simulink model "Ford_T3T6_ArchCnctnDigrm"  (R2016b)
settings: Solver=FixedStepDiscrete  StartTime=0.0  StopTime=10.0  RelTol=1e-3  EnableMultiTasking=on
libraries: canmsglib x15
(part 12 of 15)

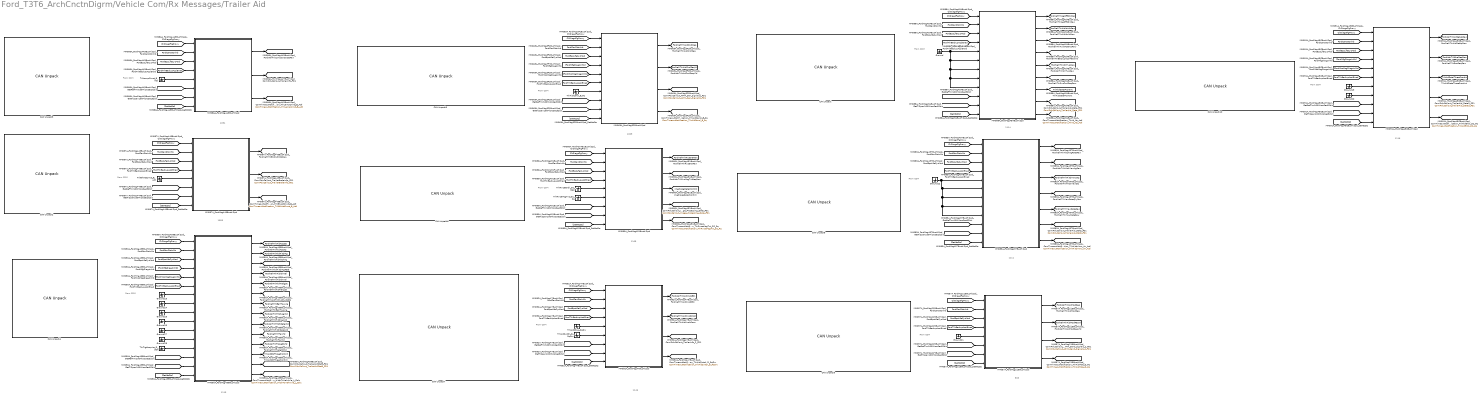
== system Ford_T3T6_ArchCnctnDigrm/Vehicle Com/Rx Messages/Trailer Aid ==
  note: 1116
  note: 533
  note: 1111
  note: 1114
  note: 1146
  note: 1105
  note: 1009
  note: 1113
  note: 1093
  note: 1091
  note: From COM
  note: From COM
  note: From COM
  note: From COM
  note: From COM
  note: From COM
  note: From COM
  note: From COM
  note: From COM
  note: From COM
  CAN Unpack : canmsglib/CAN Unpack  CANdbFile=C:\Users\nz3503\Desktop\Ford Architecture\FD1_CAN_P702_GASDHEV_MY21_V04.dbc  MsgList=TrailerAid_Data_FD1  MsgName=TrailerAid_Data_FD1  MsgIDType=Standard (11-bit identifier)  MsgIdentifier=1114  MsgLength=8  SignalInfo=TrailCtlSwtch_B_Stat2$16$1$2$2$1$0$1$0$0$1$#TrlBrkInitOut_D_Rq$59$2$2$2$1$0$1$0$0$3$#TrlrAidEnbl_D_Rq$13$2$2$2$1$0$1$0$0$3$#TrlrAidSetup_D_Rq$57$2$2$2$1$0$1$0$0$3$#TrlrAnOffstDir_D_Mem$61$2$2$2$1$0$1$0$0$3$#TrlrAnOffst_An_Mem$63$9$2$2$1$0$1.000000e-01$0$0$5.110000e+01$#TrlrAxleToBmpr_L_Actl$15$9$2$2$1$0$2.540000e-02$0$0$1.297940e+01$#TrlrBallToBmpr_L_Actl$17$7$2$2$1$0$1.270000e-02$0$0$1.612900e+00$#TrlrIdType_D_Stat$32$2$2$2$1$0$1$0$0$3$#TrlrId_No_Actl$9$4$2$2$1$0$1$0$0$15$#TrlrRvrseCancl_B_Rq$8$1$2$2$1$0$1$0$0$1$#TrlrTrgtOffst_L_Actl$41$7$2$2$1$0$1.270000e-02$0$0$1.612900e+00$#TrlrTrgtPtrnId_No_Mem$34$6$2$2$1$0$1$0$0$63$#TrlrTrgtToBmpr_L_Actl$25$7$2$2$1$0$1.270000e-02$0$0$1.612900e+00$#  NSignals=14  IDPort=off  TimestampPort=off  ErrorPort=off  RemotePort=off  LengthPort=off  StatusPort=off  StartBits=str2num('[int32(16);int32(59);int32(13);int32(57);int32(61);int32(63);int32(15);int32(17);int32(32);int32(9);int32(8);int32(41);int32(34);int32(25)]')  SignalSizes=str2num('[int32(1);int32(2);int32(2);int32(2);int32(2);int32(9);int32(9);int32(7);int32(2);int32(4);int32(1);int32(7);int32(6);int32(7)]')  ByteOrders=str2num('[int32(2);int32(2);int32(2);int32(2);int32(2);int32(2);int32(2);int32(2);int32(2);int32(2);int32(2);int32(2);int32(2);int32(2)]')  DataTypes=str2num('[int32(2);int32(2);int32(2);int32(2);int32(2);int32(2);int32(2);int32(2);int32(2);int32(2);int32(2);int32(2);int32(2);int32(2)]')  MultiplexTypes=str2num('[int32(1);int32(1);int32(1);int32(1);int32(1);int32(1);int32(1);int32(1);int32(1);int32(1);int32(1);int32(1);int32(1);int32(1)]')  MultiplexValues=str2num('[double(0);double(0);double(0);double(0);double(0);double(0);double(0);double(0);double(0);double(0);double(0);double(0);double(0);double(0)]')  Factors=str2num('[double(1);double(1);double(1);double(1);double(1);double(1.000000e-01);double(2.540000e-02);double(1.270000e-02);double(1);double(1);double(1);double(1.270000e-02);double(1);double(1.270000e-02)]')  Offsets=str2num('[double(0);double(0);double(0);double(0);double(0);double(0);double(0);double(0);double(0);double(0);double(0);double(0);double(0);double(0)]')  Minimums=str2num('[double(0);double(0);double(0);double(0);double(0);double(0);double(0);double(0);double(0);double(0);double(0);double(0);double(0);double(0)]')  Maximums=str2num('[double(1);double(3);double(3);double(3);double(3);double(5.110000e+01);double(1.297940e+01);double(1.612900e+00);double(3);double(15);double(1);double(1.612900e+00);double(63);double(1.612900e+00)]')
      settings: DataFormat=CANdb specified signals
  CAN Unpack10 : canmsglib/CAN Unpack  CANdbFile=C:\Users\nz3503\Desktop\Ford Architecture\FD1_CAN_P702_GASDHEV_MY21_V04.dbc  MsgList=TrailerAid_Data3_FD1  MsgName=TrailerAid_Data3_FD1  MsgIDType=Standard (11-bit identifier)  MsgIdentifier=1116  MsgLength=8  SignalInfo=TrlrAidEnbl_D2_Rq$5$3$2$2$1$0$1$0$0$7$#TrlrAidSetup_D2_Rq$1$4$2$2$1$0$1$0$0$15$#  NSignals=2  IDPort=off  TimestampPort=off  ErrorPort=off  RemotePort=off  LengthPort=off  StatusPort=off  StartBits=str2num('[int32(5);int32(1)]')  SignalSizes=str2num('[int32(3);int32(4)]')  ByteOrders=str2num('[int32(2);int32(2)]')  DataTypes=str2num('[int32(2);int32(2)]')  MultiplexTypes=str2num('[int32(1);int32(1)]')  MultiplexValues=str2num('[double(0);double(0)]')  Factors=str2num('[double(1);double(1)]')  Offsets=str2num('[double(0);double(0)]')  Minimums=str2num('[double(0);double(0)]')  Maximums=str2num('[double(7);double(15)]')
      settings: DataFormat=CANdb specified signals
  CAN Unpack2 : canmsglib/CAN Unpack  CANdbFile=C:\Users\nz3503\Desktop\Ford Architecture\FD1_CAN_P702_GASDHEV_MY21_V04.dbc  MsgList=TrailerBrakeInfo_FD1  MsgName=TrailerBrakeInfo_FD1  MsgIDType=Standard (11-bit identifier)  MsgIdentifier=1093  MsgLength=8  SignalInfo=StopLamp_B_RqTrlrBrk$7$1$2$2$1$0$1$0$0$1$#TrlBrkInitOut_D_Stat$9$2$2$2$1$0$1$0$0$3$#TrlrBrkActCirct_B_Falt$1$1$2$2$1$0$1$0$0$1$#TrlrBrkActCnnct_B_Actl$6$1$2$2$1$0$1$0$0$1$#TrlrBrkCtl_B_Falt$4$1$2$2$1$0$1$0$0$1$#TrlrBrkDcnnt_B_Actl$5$1$2$2$1$0$1$0$0$1$#TrlrBrkDsply_B_Rq$3$1$2$2$1$0$1$0$0$1$#TrlrBrkGain_No_Actl$11$5$2$2$1$0$5.000000e-01$0$0$1.550000e+01$#TrlrBrkMde_D_Actl$2$1$2$2$1$0$1$0$0$1$#TrlrBrkOut_No_Dsply$20$4$2$2$1$0$1$0$0$15$#  NSignals=10  IDPort=off  TimestampPort=off  ErrorPort=off  RemotePort=off  LengthPort=off  StatusPort=off  StartBits=str2num('[int32(7);int32(9);int32(1);int32(6);int32(4);int32(5);int32(3);int32(11);int32(2);int32(20)]')  SignalSizes=str2num('[int32(1);int32(2);int32(1);int32(1);int32(1);int32(1);int32(1);int32(5);int32(1);int32(4)]')  ByteOrders=str2num('[int32(2);int32(2);int32(2);int32(2);int32(2);int32(2);int32(2);int32(2);int32(2);int32(2)]')  DataTypes=str2num('[int32(2);int32(2);int32(2);int32(2);int32(2);int32(2);int32(2);int32(2);int32(2);int32(2)]')  MultiplexTypes=str2num('[int32(1);int32(1);int32(1);int32(1);int32(1);int32(1);int32(1);int32(1);int32(1);int32(1)]')  MultiplexValues=str2num('[double(0);double(0);double(0);double(0);double(0);double(0);double(0);double(0);double(0);double(0)]')  Factors=str2num('[double(1);double(1);double(1);double(1);double(1);double(1);double(1);double(5.000000e-01);double(1);double(1)]')  Offsets=str2num('[double(0);double(0);double(0);double(0);double(0);double(0);double(0);double(0);double(0);double(0)]')  Minimums=str2num('[double(0);double(0);double(0);double(0);double(0);double(0);double(0);double(0);double(0);double(0)]')  Maximums=str2num('[double(1);double(3);double(1);double(1);double(1);double(1);double(1);double(1.550000e+01);double(1);double(15)]')
      settings: DataFormat=CANdb specified signals
  CAN Unpack3 : canmsglib/CAN Unpack  CANdbFile=C:\Users\nz3503\Desktop\Ford Architecture\FD1_CAN_P702_GASDHEV_MY21_V04.dbc  MsgList=TrailerInfo_FD1  MsgName=TrailerInfo_FD1  MsgIDType=Standard (11-bit identifier)  MsgIdentifier=1091  MsgLength=8  SignalInfo=CamraRearOn_D2_Stat2$9$3$2$2$1$0$1$0$0$7$#ParkLampTrlrOut_B_Stat$15$1$2$2$1$0$1$0$0$1$#PoliceAux1Lamp_B_Rq2$8$1$2$2$1$0$1$0$0$1$#PoliceAux2Lamp_B_Rq2$23$1$2$2$1$0$1$0$0$1$#PoliceAux3Lamp_B_Rq2$22$1$2$2$1$0$1$0$0$1$#PoliceAux4Lamp_B_Rq2$21$1$2$2$1$0$1$0$0$1$#StopLampTrlrOut_B_Stat$0$1$2$2$1$0$1$0$0$1$#TowBarMsgTxt_D_Rq$12$3$2$2$1$0$1$0$0$7$#TrlrBattChrg_D_Stat$1$2$2$2$1$0$1$0$0$3$#TrlrLampCnnct_B_Actl$7$1$2$2$1$0$1$0$0$1$#TrlrLampCtl_D_Stat$3$2$2$2$1$0$1$0$0$3$#TurnLampTrlrRl_B_Stat$6$1$2$2$1$0$1$0$0$1$#TurnLampTrlrRr_B_Stat$5$1$2$2$1$0$1$0$0$1$#  NSignals=13  IDPort=off  TimestampPort=off  ErrorPort=off  RemotePort=off  LengthPort=off  StatusPort=off  StartBits=str2num('[int32(9);int32(15);int32(8);int32(23);int32(22);int32(21);int32(0);int32(12);int32(1);int32(7);int32(3);int32(6);int32(5)]')  SignalSizes=str2num('[int32(3);int32(1);int32(1);int32(1);int32(1);int32(1);int32(1);int32(3);int32(2);int32(1);int32(2);int32(1);int32(1)]')  ByteOrders=str2num('[int32(2);int32(2);int32(2);int32(2);int32(2);int32(2);int32(2);int32(2);int32(2);int32(2);int32(2);int32(2);int32(2)]')  DataTypes=str2num('[int32(2);int32(2);int32(2);int32(2);int32(2);int32(2);int32(2);int32(2);int32(2);int32(2);int32(2);int32(2);int32(2)]')  MultiplexTypes=str2num('[int32(1);int32(1);int32(1);int32(1);int32(1);int32(1);int32(1);int32(1);int32(1);int32(1);int32(1);int32(1);int32(1)]')  MultiplexValues=str2num('[double(0);double(0);double(0);double(0);double(0);double(0);double(0);double(0);double(0);double(0);double(0);double(0);double(0)]')  Factors=str2num('[double(1);double(1);double(1);double(1);double(1);double(1);double(1);double(1);double(1);double(1);double(1);double(1);double(1)]')  Offsets=str2num('[double(0);double(0);double(0);double(0);double(0);double(0);double(0);double(0);double(0);double(0);double(0);double(0);double(0)]')  Minimums=str2num('[double(0);double(0);double(0);double(0);double(0);double(0);double(0);double(0);double(0);double(0);double(0);double(0);double(0)]')  Maximums=str2num('[double(7);double(1);double(1);double(1);double(1);double(1);double(1);double(7);double(3);double(1);double(3);double(1);double(1)]')
      settings: DataFormat=CANdb specified signals
  CAN Unpack4 : canmsglib/CAN Unpack  CANdbFile=C:\Users\nz3503\Desktop\Ford Architecture\FD1_CAN_P702_GASDHEV_MY21_V04.dbc  MsgList=TrailerAid_Stat3_FD1  MsgName=TrailerAid_Stat3_FD1  MsgIDType=Standard (11-bit identifier)  MsgIdentifier=1113  MsgLength=8  SignalInfo=HitchToTrlrAxle_L_Calc2$23$9$2$2$1$0$2.540000e-02$0$0$1.297940e+01$#HitchToVehAxle_L_Calc$0$8$2$2$1$0$1.270000e-02$-5.080000e-01$-5.080000e-01$2.717800e+00$#TrlrAidTrgtId_No_Actl$43$5$2$2$1$0$1$0$0$31$#TrlrAid_An3_Actl$34$11$2$2$1$0$1.250000e-01$-90$-90$1.657500e+02$#TrlrAid_AnRate2_Actl$29$10$2$2$1$0$1.250000e-01$-50$-50$7.775000e+01$#TrlrAid_D2_Stat$52$4$2$2$1$0$1$0$0$15$#TrlrAnCalib_B_Complt$40$1$2$2$1$0$1$0$0$1$#TrlrAnOffstDir_D_Calc$32$2$2$2$1$0$1$0$0$3$#TrlrAnOffst_An_Calc$56$9$2$2$1$0$1.000000e-01$0$0$5.110000e+01$#TrlrRvrse_D_Stat$41$2$2$2$1$0$1$0$0$3$#TrlrTrgtAcquire_D_Stat$49$3$2$2$1$0$1$0$0$7$#  NSignals=11  IDPort=off  TimestampPort=off  ErrorPort=off  RemotePort=off  LengthPort=off  StatusPort=off  StartBits=str2num('[int32(23);int32(0);int32(43);int32(34);int32(29);int32(52);int32(40);int32(32);int32(56);int32(41);int32(49)]')  SignalSizes=str2num('[int32(9);int32(8);int32(5);int32(11);int32(10);int32(4);int32(1);int32(2);int32(9);int32(2);int32(3)]')  ByteOrders=str2num('[int32(2);int32(2);int32(2);int32(2);int32(2);int32(2);int32(2);int32(2);int32(2);int32(2);int32(2)]')  DataTypes=str2num('[int32(2);int32(2);int32(2);int32(2);int32(2);int32(2);int32(2);int32(2);int32(2);int32(2);int32(2)]')  MultiplexTypes=str2num('[int32(1);int32(1);int32(1);int32(1);int32(1);int32(1);int32(1);int32(1);int32(1);int32(1);int32(1)]')  MultiplexValues=str2num('[double(0);double(0);double(0);double(0);double(0);double(0);double(0);double(0);double(0);double(0);double(0)]')  Factors=str2num('[double(2.540000e-02);double(1.270000e-02);double(1);double(1.250000e-01);double(1.250000e-01);double(1);double(1);double(1);double(1.000000e-01);double(1);double(1)]')  Offsets=str2num('[double(0);double(-5.080000e-01);double(0);double(-90);double(-50);double(0);double(0);double(0);double(0);double(0);double(0)]')  Minimums=str2num('[double(0);double(-5.080000e-01);double(0);double(-90);double(-50);double(0);double(0);double(0);double(0);double(0);double(0)]')  Maximums=str2num('[double(1.297940e+01);double(2.717800e+00);double(31);double(1.657500e+02);double(7.775000e+01);double(15);double(1);double(3);double(5.110000e+01);double(3);double(7)]')
      settings: DataFormat=CANdb specified signals
  CAN Unpack5 : canmsglib/CAN Unpack  CANdbFile=C:\Users\nz3503\Desktop\Ford Architecture\FD1_CAN_P702_GASDHEV_MY21_V04.dbc  MsgList=APIM_Send_Signals1_FD1  MsgName=APIM_Send_Signals1_FD1  MsgIDType=Standard (11-bit identifier)  MsgIdentifier=1009  MsgLength=8  SignalInfo=APIM_ActiveTrackNum_St$24$32$2$2$1$0$1$0$0$4294967295$#APIM_NumberofTracks_St$40$16$2$2$1$0$1$0$0$65535$#AutoHoldSwtch_D_Stat3$49$2$2$2$1$0$1$0$0$3$#CenterStackRing_D_Actl$58$2$2$2$1$0$1$0$0$3$#ChrgCordUnlock_B_Rq$60$1$2$2$1$0$1$0$0$1$#TrlrAidCancl_B_Rq$48$1$2$2$1$0$1$0$0$1$#TrlrAidSetup_D_Stat$53$3$2$2$1$0$1$0$0$7$#TrlrTrgtAcquire_D_Rq$61$3$2$2$1$0$1$0$0$7$#ValetMode_D_Stat$56$2$2$2$1$0$1$0$0$3$#  NSignals=9  IDPort=off  TimestampPort=off  ErrorPort=off  RemotePort=off  LengthPort=off  StatusPort=off  StartBits=str2num('[int32(24);int32(40);int32(49);int32(58);int32(60);int32(48);int32(53);int32(61);int32(56)]')  SignalSizes=str2num('[int32(32);int32(16);int32(2);int32(2);int32(1);int32(1);int32(3);int32(3);int32(2)]')  ByteOrders=str2num('[int32(2);int32(2);int32(2);int32(2);int32(2);int32(2);int32(2);int32(2);int32(2)]')  DataTypes=str2num('[int32(2);int32(2);int32(2);int32(2);int32(2);int32(2);int32(2);int32(2);int32(2)]')  MultiplexTypes=str2num('[int32(1);int32(1);int32(1);int32(1);int32(1);int32(1);int32(1);int32(1);int32(1)]')  MultiplexValues=str2num('[double(0);double(0);double(0);double(0);double(0);double(0);double(0);double(0);double(0)]')  Factors=str2num('[double(1);double(1);double(1);double(1);double(1);double(1);double(1);double(1);double(1)]')  Offsets=str2num('[double(0);double(0);double(0);double(0);double(0);double(0);double(0);double(0);double(0)]')  Minimums=str2num('[double(0);double(0);double(0);double(0);double(0);double(0);double(0);double(0);double(0)]')  Maximums=str2num('[double(4294967295);double(65535);double(3);double(3);double(1);double(1);double(7);double(7);double(3)]')
      settings: DataFormat=CANdb specified signals
  CAN Unpack6 : canmsglib/CAN Unpack  CANdbFile=C:\Users\nz3503\Desktop\Ford Architecture\FD1_CAN_P702_GASDHEV_MY21_V04.dbc  MsgList=Image_Processing_Data_FD1  MsgName=Image_Processing_Data_FD1  MsgIDType=Standard (11-bit identifier)  MsgIdentifier=1105  MsgLength=8  SignalInfo=BrkDecel_B_RqRba$8$1$2$2$1$0$1$0$0$1$#BrkEnbl_B_RqRba$23$1$2$2$1$0$1$0$0$1$#CamraFrntStat_D_Stat$6$2$2$2$1$0$1$0$0$3$#CamraRemoteStat_B_Actl$5$1$2$2$1$0$1$0$0$1$#RbaAlrt_D_Dsply$11$2$2$2$1$0$1$0$0$3$#RbaMnu_D_Rq$9$2$2$2$1$0$1$0$0$3$#RbaMsg_D_Rq$21$2$2$2$1$0$1$0$0$3$#RbaSys_D_Stat$19$2$2$2$1$0$1$0$0$3$#Rba_D_Stat$13$2$2$2$1$0$1$0$0$3$#TrlrHitchLamp_D_Rq2$15$1$2$2$1$0$1$0$0$1$#TrlrRvrseEnbl_D2_Stat$16$3$2$2$1$0$1$0$0$7$#TrlrRvrseMsgTxt_D2_Rq$26$6$2$2$1$0$1$0$0$63$#TrlrRvrseMsgTxt_D_Rq$0$5$2$2$1$0$1$0$0$31$#  NSignals=13  IDPort=off  TimestampPort=off  ErrorPort=off  RemotePort=off  LengthPort=off  StatusPort=off  StartBits=str2num('[int32(8);int32(23);int32(6);int32(5);int32(11);int32(9);int32(21);int32(19);int32(13);int32(15);int32(16);int32(26);int32(0)]')  SignalSizes=str2num('[int32(1);int32(1);int32(2);int32(1);int32(2);int32(2);int32(2);int32(2);int32(2);int32(1);int32(3);int32(6);int32(5)]')  ByteOrders=str2num('[int32(2);int32(2);int32(2);int32(2);int32(2);int32(2);int32(2);int32(2);int32(2);int32(2);int32(2);int32(2);int32(2)]')  DataTypes=str2num('[int32(2);int32(2);int32(2);int32(2);int32(2);int32(2);int32(2);int32(2);int32(2);int32(2);int32(2);int32(2);int32(2)]')  MultiplexTypes=str2num('[int32(1);int32(1);int32(1);int32(1);int32(1);int32(1);int32(1);int32(1);int32(1);int32(1);int32(1);int32(1);int32(1)]')  MultiplexValues=str2num('[double(0);double(0);double(0);double(0);double(0);double(0);double(0);double(0);double(0);double(0);double(0);double(0);double(0)]')  Factors=str2num('[double(1);double(1);double(1);double(1);double(1);double(1);double(1);double(1);double(1);double(1);double(1);double(1);double(1)]')  Offsets=str2num('[double(0);double(0);double(0);double(0);double(0);double(0);double(0);double(0);double(0);double(0);double(0);double(0);double(0)]')  Minimums=str2num('[double(0);double(0);double(0);double(0);double(0);double(0);double(0);double(0);double(0);double(0);double(0);double(0);double(0)]')  Maximums=str2num('[double(1);double(1);double(3);double(1);double(3);double(3);double(3);double(3);double(3);double(1);double(7);double(63);double(31)]')
      settings: DataFormat=CANdb specified signals
  CAN Unpack7 : canmsglib/CAN Unpack  CANdbFile=C:\Users\nz3503\Desktop\Ford Architecture\FD1_CAN_P702_GASDHEV_MY21_V04.dbc  MsgList=TrailerInfo_2_FD1  MsgName=TrailerInfo_2_FD1  MsgIDType=Standard (11-bit identifier)  MsgIdentifier=1146  MsgLength=8  SignalInfo=TrlrAidAn_URate_Actl$16$12$2$2$1$0$1.250000e-03$-2.500000e+00$-2.500000e+00$2.616250e+00$#TrlrAidAn_U_Actl$12$12$2$2$1$0$1.250000e-03$0$0$5.116250e+00$#TrlrAidCtl_U_RqDrv$36$12$2$2$1$0$1.250000e-03$0$0$5.116250e+00$#TrlrAidSwtch_D_RqDrv$34$2$2$2$1$0$1$0$0$3$#  NSignals=4  IDPort=off  TimestampPort=off  ErrorPort=off  RemotePort=off  LengthPort=off  StatusPort=off  StartBits=str2num('[int32(16);int32(12);int32(36);int32(34)]')  SignalSizes=str2num('[int32(12);int32(12);int32(12);int32(2)]')  ByteOrders=str2num('[int32(2);int32(2);int32(2);int32(2)]')  DataTypes=str2num('[int32(2);int32(2);int32(2);int32(2)]')  MultiplexTypes=str2num('[int32(1);int32(1);int32(1);int32(1)]')  MultiplexValues=str2num('[double(0);double(0);double(0);double(0)]')  Factors=str2num('[double(1.250000e-03);double(1.250000e-03);double(1.250000e-03);double(1)]')  Offsets=str2num('[double(-2.500000e+00);double(0);double(0);double(0)]')  Minimums=str2num('[double(-2.500000e+00);double(0);double(0);double(0)]')  Maximums=str2num('[double(2.616250e+00);double(5.116250e+00);double(5.116250e+00);double(3)]')
      settings: DataFormat=CANdb specified signals
  CAN Unpack8 : canmsglib/CAN Unpack  CANdbFile=C:\Users\nz3503\Desktop\Ford Architecture\FD1_CAN_P702_GASDHEV_MY21_V04.dbc  MsgList=TrailerAid_Stat2_FD1  MsgName=TrailerAid_Stat2_FD1  MsgIDType=Standard (11-bit identifier)  MsgIdentifier=1111  MsgLength=8  SignalInfo=TrlrHitYaw_AnRate_Actl$32$12$2$2$1$0$1.000000e-01$-50$-50$3.593000e+02$#TrlrHitchYaw_An_Actl$28$12$2$2$1$0$1.000000e-01$-90$-90$3.193000e+02$#TrlrHitchYaw_D_Stat$44$4$2$2$1$0$1$0$0$15$#TrlrYawWActl_D_Qf$42$2$2$2$1$0$1$0$0$3$#TrlrYaw_W_Actl$8$16$2$2$1$0$2.000000e-04$-6.500000e+00$-6.500000e+00$6.606600e+00$#  NSignals=5  IDPort=off  TimestampPort=off  ErrorPort=off  RemotePort=off  LengthPort=off  StatusPort=off  StartBits=str2num('[int32(32);int32(28);int32(44);int32(42);int32(8)]')  SignalSizes=str2num('[int32(12);int32(12);int32(4);int32(2);int32(16)]')  ByteOrders=str2num('[int32(2);int32(2);int32(2);int32(2);int32(2)]')  DataTypes=str2num('[int32(2);int32(2);int32(2);int32(2);int32(2)]')  MultiplexTypes=str2num('[int32(1);int32(1);int32(1);int32(1);int32(1)]')  MultiplexValues=str2num('[double(0);double(0);double(0);double(0);double(0)]')  Factors=str2num('[double(1.000000e-01);double(1.000000e-01);double(1);double(1);double(2.000000e-04)]')  Offsets=str2num('[double(-50);double(-90);double(0);double(0);double(-6.500000e+00)]')  Minimums=str2num('[double(-50);double(-90);double(0);double(0);double(-6.500000e+00)]')  Maximums=str2num('[double(3.593000e+02);double(3.193000e+02);double(15);double(3);double(6.606600e+00)]')
      settings: DataFormat=CANdb specified signals
  CAN Unpack9 : canmsglib/CAN Unpack  CANdbFile=C:\Users\nz3503\Desktop\Ford Architecture\FD1_CAN_P702_GASDHEV_MY21_V04.dbc  MsgList=APIM_Send_Signals_2_FD1  MsgName=APIM_Send_Signals_2_FD1  MsgIDType=Standard (11-bit identifier)  MsgIdentifier=533  MsgLength=8  SignalInfo=OnbChrgClearAll_B_Rq$18$1$2$2$1$0$1$0$0$1$#OnbChrgGoTDelete_B_Rq$17$1$2$2$1$0$1$0$0$1$#OnbChrgGoTElement_D_Rq$28$4$2$2$1$0$1$0$0$15$#OnbChrgGoTExtHtr_D_Rq$26$2$2$2$1$0$1$0$0$3$#OnbChrgGoTHr_T_Rq$35$5$2$2$1$0$1$0$0$29$#OnbChrgGoTMnte_D_Rq$44$4$2$2$1$0$1$0$0$15$#OnbChrgGoTOn_D_Rq$24$2$2$2$1$0$1$0$0$3$#OnbChrgGoTPrcond_D_Rq$33$2$2$2$1$0$1$0$0$3$#OnbChrgGoTTouch_D_Rq$42$2$2$2$1$0$1$0$0$3$#OnbChrgGoTUpdate_B_Rq$16$1$2$2$1$0$1$0$0$1$#OtaTrg_D_Stat$40$2$2$2$1$0$1$0$0$3$#PaakMyKey_D_Rq$6$2$2$2$1$0$1$0$0$3$#TCU_Final_Actvtn_St$2$2$2$2$1$0$1$0$0$3$#TCU_Init_Actvtn_St$0$2$2$2$1$0$1$0$0$3$#TrlrAidMde_D_Rq$4$2$2$2$1$0$1$0$0$3$#  NSignals=15  IDPort=off  TimestampPort=off  ErrorPort=off  RemotePort=off  LengthPort=off  StatusPort=off  StartBits=str2num('[int32(18);int32(17);int32(28);int32(26);int32(35);int32(44);int32(24);int32(33);int32(42);int32(16);int32(40);int32(6);int32(2);int32(0);int32(4)]')  SignalSizes=str2num('[int32(1);int32(1);int32(4);int32(2);int32(5);int32(4);int32(2);int32(2);int32(2);int32(1);int32(2);int32(2);int32(2);int32(2);int32(2)]')  ByteOrders=str2num('[int32(2);int32(2);int32(2);int32(2);int32(2);int32(2);int32(2);int32(2);int32(2);int32(2);int32(2);int32(2);int32(2);int32(2);int32(2)]')  DataTypes=str2num('[int32(2);int32(2);int32(2);int32(2);int32(2);int32(2);int32(2);int32(2);int32(2);int32(2);int32(2);int32(2);int32(2);int32(2);int32(2)]')  MultiplexTypes=str2num('[int32(1);int32(1);int32(1);int32(1);int32(1);int32(1);int32(1);int32(1);int32(1);int32(1);int32(1);int32(1);int32(1);int32(1);int32(1)]')  MultiplexValues=str2num('[double(0);double(0);double(0);double(0);double(0);double(0);double(0);double(0);double(0);double(0);double(0);double(0);double(0);double(0);double(0)]')  Factors=str2num('[double(1);double(1);double(1);double(1);double(1);double(1);double(1);double(1);double(1);double(1);double(1);double(1);double(1);double(1);double(1)]')  Offsets=str2num('[double(0);double(0);double(0);double(0);double(0);double(0);double(0);double(0);double(0);double(0);double(0);double(0);double(0);double(0);double(0)]')  Minimums=str2num('[double(0);double(0);double(0);double(0);double(0);double(0);double(0);double(0);double(0);double(0);double(0);double(0);double(0);double(0);double(0)]')  Maximums=str2num('[double(1);double(1);double(15);double(3);double(29);double(15);double(3);double(3);double(3);double(1);double(3);double(3);double(3);double(3);double(3)]')
      settings: DataFormat=CANdb specified signals
  Ground{,19..28} (11 alike) : Ground
  MM057A_FordMsg215BusHiSpd : Subsystem  Tag=4.0.X  Description=The purpose of the Ford Message 215 Bus High Speed function is to provide the Electric Power Steering system with Trailer Back up Assist and Gear Lever Position signals from CAN. The Ford Message 215 function will perform the missing message and signal invalid diagnostics as well as provide a validity signal for the signal values and received message
      settings: AttributesFormatString=Version: %<Tag>
  MM069A_FordMsg3F1BusHiSpd : Subsystem  Tag=4.0.X  Description=The purpose of the Ford Message 3F1 Bus High Speed function is to provide the Electric Power Steering system with vehicle odometer, climate, and Trailer Back Up Assist signals from CAN. The Ford Message 3F1 function will perform the missing message and signal invalid diagnostics as well as provide a validity signal for the signal values and received message.
      settings: AttributesFormatString=Version: %<Tag>
  MM080A_FordMsg451BusHiSpd : Subsystem  Tag=4.0.X  Description=The purpose of the Ford Message 451 Bus High Speed function is to provide the Electric Power Steering system with signal values for the Trailer Back Up Assist and Electric Power Steering functions from CAN. The Ford Message 451 function will perform the missing message and signal invalid diagnostic as well as provide a validity signal for the received message. Detailed requirements have implemented the Ford DBC file for guidance.
      settings: AttributesFormatString=Version: %<Tag>
  MM083A_FordMsg457BusHiSpd : Subsystem  Tag=4.0.X  Description=The purpose of the Ford Message 457 Bus High Speed function is to provide the Electric Power Steering system with Trailer Back up Assist and Gear Lever Position signals from CAN. The Ford Message 457 function will perform the missing message and signal invalid diagnostics as well as provide a validity signal for the signal values and received message
      settings: AttributesFormatString=Version: %<Tag>
  MM086A_FordMsg443BusHiSpd : Subsystem  Tag=4.0.X  Description=The purpose of the Ford Message 443 Bus High Speed function is to provide the Electric Power Steering system with signal values for the Trailer Back Up Assist function from CAN. The Ford Message 443 function will perform the missing message diagnostic.
      settings: AttributesFormatString=Version: %<Tag>
  MM087A_FordMsg445BusHiSpd : Subsystem  Tag=4.0.X  Description=The purpose of the Ford Message 445 Bus High Speed function is to provide the Electric Power Steering system with signal values for the Trailer Back Up Assist function from CAN. The Ford Message 445 function will perform the missing message diagnostic. Detailed requirements have implemented the Ford DBC file for guidance.
      settings: AttributesFormatString=Version: %<Tag>
  MM088A_FordMsg45ABusHiSpd : Subsystem  Tag=4.0.X  Description=The purpose of the Ford Message 45A Bus High Speedfunction is to provide the Electric Power Steeringsystem with signal values for the Trailer Back UpAssist function from CAN. The Ford Message 45A functionwill perform the missing message as well as provide avalidity signal for the received message
      settings: AttributesFormatString=Version: %<Tag>
  MM090A_FordMsg459BusHiSpd : Subsystem  Tag=0.0.X
      settings: AttributesFormatString=Version: %<Tag>
  MM091A_FordMsg45CBusHiSpd : Subsystem  Tag=0.0.X
      settings: AttributesFormatString=Version: %<Tag>
  MM092A_FordMsg47BusHiSpd : Subsystem  Tag=4.0.X  Description=The purpose of the Ford Message 47A Bus High Speed function is to providethe Electric Power Steering system with signal values for the Trailer Back UpAssist and Electric Power Steering functions from CAN. The Ford Message 47Afunction will perform the missing message and signal invalid diagnostic as wellas provide a validity signal for the received message.
      settings: AttributesFormatString=Version: %<Tag>
  TrlrAidCancl_B_Rq : Ground
  TrlrAidCtl_U_RqDrv : Ground
  TrlrAidSwtch_D_RqDrv : Ground
  TrlrBrkActCnnct_B_Actl : Ground
  TrlrLampCnnct_B_Actl : Ground
  TrlrRvrseEnbl_D2_Stat : Ground
  TrlrRvrseMsgTxt_D2_Rq : Ground
  TrlrTrgtAcquire_D_Stat : Ground
  tag scope: ComIPduCallout_APIM_Sen_Signals1_FD1=global, ComIPduCallout_APIM_Send_Signals_2_FD1=global, ComIPduCallout_Image_Processing_Data_FD1=global, ComIPduCallout_TrailerAidStat3_FD1=global, ComIPduCallout_TrailerAid_Data3_FD1=global, ComIPduCallout_TrailerAid_Data_FD1=global, ComIPduCallout_TrailerAid_Stat2_FD1=global, ComIPduCallout_TrailerBrakeInfo_FD1=global, ComIPduCallout_TrailerInfo_2_FD1=global, ComIPduCallout_TrailerInfo_FD1=global, ComTimeoutNotification_HitchToVehAxle_L_Calc=global, ComTimeoutNotification_TrlrAidCancl_B_Rq=global, ComTimeoutNotification_TrlrAidEnbl_D2_Rq=global, ComTimeoutNotification_TrlrAidMde_D_Rq=global, ComTimeoutNotification_TrlrAidSwtch_D_RqDrv=global, ComTimeoutNotification_TrlrBrkActCnnct_B_Actl=global, ComTimeoutNotification_TrlrHitchYaw_An_Actl=global, ComTimeoutNotification_TrlrId_No_Actl=global, ComTimeoutNotification_TrlrLampCnnct_B_Actl=global, ComTimeoutNotification_TrlrRvrseMsgTxt_D2_Rq=global, FordVehTrlrAgOffsDirRaw=global, FordVehTrlrAidAcqSts=global, FordVehTrlrAidCnclReq=global, FordVehTrlrAidCnclReqVld=global, FordVehTrlrAidHitchAg=global, FordVehTrlrAidHitchAgRate=global, FordVehTrlrAidIdnNrRaw=global, FordVehTrlrAidIdnVal=global, FordVehTrlrAidKnobBtn=global, FordVehTrlrAidKnobPosn=global, FordVehTrlrAidModReq=global, FordVehTrlrAidModReqVld=global, FordVehTrlrAidSetUpRaw=global, FordVehTrlrAidTrakgSt=global, FordVehTrlrAidTrlrRvsGuidcSts=global, FordVehTrlrAxleToBmpRaw=global, FordVehTrlrBackupAssiMeasVld=global, FordVehTrlrBallToAxle=global, FordVehTrlrBrkCnctnStsRaw=global, FordVehTrlrEnaReqRaw=global, FordVehTrlrHitchAgRateRaw=global, FordVehTrlrHitchAgVld=global, FordVehTrlrHitchRateVld=global, FordVehTrlrHitchYawAgRaw=global, FordVehTrlrHitchYawSts=global, FordVehTrlrIdnTypRaw=global, FordVehTrlrLampCnctnStsRaw=global, FordVehTrlrRvsCnclReqRaw=global, FordVehTrlrRvsEnaRaw=global, FordVehTrlrRvsMsgTxtReqRaw=global, FordVehTrlrTarVld=global, FordVehTrlrTrakgStVld=global, FordVehTrlrYawRateQlyFac=global, FordVehTrlrYawRateRaw=global, ImgProcgDataPrsntInt=global, TrlrAidDataPrsntInt=global, TrlrAidDataThreePrsntInt=global, TrlrAidStsThreePrsntInt=global
  wires:
  [ClrDiagcFlgProxy] -> MM091A_FordMsg45CBusHiSpd/1(ClrDiagcFlgProxy)
  [FordCanDtcInhb] -> MM091A_FordMsg45CBusHiSpd/2(FordCanDtcInhb)
  [FordEpsLifeCycMod] -> MM091A_FordMsg45CBusHiSpd/3(FordEpsLifeCycMod)
  [FordMfgDiagcInhb] -> MM091A_FordMsg45CBusHiSpd/4(FordMfgDiagcInhb)
  [FordMissMsgDiagcInhb] -> MM091A_FordMsg45CBusHiSpd/5(FordMissMsgDiagcInhb)
  [FordTrlrBackupAssiEnad] -> MM091A_FordMsg45CBusHiSpd/6(FordTrlrBackupAssiEnad)
  Ground19/1 -> MM091A_FordMsg45CBusHiSpd/7(Ford_TrlrAidEnbl_D2_Rq)
  Ground20/1 -> MM091A_FordMsg45CBusHiSpd/8(Ford_TrlrAidSetup_D2_Rq)
  [GetRefTmr100MicroSec32bit] -> MM091A_FordMsg45CBusHiSpd/9(GetRefTmr100MicroSec32bit)
  [GetTiSpan100MicroSec32bit] -> MM091A_FordMsg45CBusHiSpd/10(GetTiSpan100MicroSec32bit)
  [SetNtcSts] -> MM091A_FordMsg45CBusHiSpd/11(SetNtcSts)
  MM091A_FordMsg45CBusHiSpd/1(FordVehTrlrAidSetUpRaw) -> [FordVehTrlrAidSetUpRaw]
  MM091A_FordMsg45CBusHiSpd/2(FordVehTrlrEnaReqRaw) -> [FordVehTrlrEnaReqRaw]
  MM091A_FordMsg45CBusHiSpd/3(TrlrAidDataThreePrsntInt) -> [TrlrAidDataThreePrsntInt]
  MM091A_FordMsg45CBusHiSpd/4(ComIPduCallout_TrailerAid_Data3_FD1) -> [ComIPduCallout_TrailerAid_Data3_FD1]
  MM091A_FordMsg45CBusHiSpd/5(ComTimeoutNotification_TrlrAidEnbl_D2_Rq) -> [ComTimeoutNotification_TrlrAidEnbl_D2_Rq]
  [ClrDiagcFlgProxy] -> MM090A_FordMsg459BusHiSpd/1(ClrDiagcFlgProxy)
  [FordCanDtcInhb] -> MM090A_FordMsg459BusHiSpd/2(FordCanDtcInhb)
  [FordEpsLifeCycMod] -> MM090A_FordMsg459BusHiSpd/3(FordEpsLifeCycMod)
  [FordMfgDiagcInhb] -> MM090A_FordMsg459BusHiSpd/4(FordMfgDiagcInhb)
  [FordMissMsgDiagcInhb] -> MM090A_FordMsg459BusHiSpd/5(FordMissMsgDiagcInhb)
  [FordTrlrBackupAssiEnad] -> MM090A_FordMsg459BusHiSpd/6(FordTrlrBackupAssiEnad)
  Ground23/1 -> MM090A_FordMsg459BusHiSpd/7(Ford_HitchToVehAxle_L_Calc)
  Ground24/1 -> MM090A_FordMsg459BusHiSpd/8(Ford_TrlrAidTrgtId_No_Actl)
  Ground25/1 -> MM090A_FordMsg459BusHiSpd/9(Ford_TrlrAid_An3_Actl)
  Ground26/1 -> MM090A_FordMsg459BusHiSpd/10(Ford_TrlrAid_AnRate2_Actl)
  Ground27/1 -> MM090A_FordMsg459BusHiSpd/11(Ford_TrlrAid_D2_Stat)
  Ground28/1 -> MM090A_FordMsg459BusHiSpd/12(Ford_TrlrRvrse_D_Stat)
  TrlrTrgtAcquire_D_Stat/1 -> MM090A_FordMsg459BusHiSpd/13(Ford_TrlrTrgtAcquire_D_Stat)
  [GetRefTmr100MicroSec32bit] -> MM090A_FordMsg459BusHiSpd/14(GetRefTmr100MicroSec32bit)
  [GetTiSpan100MicroSec32bit] -> MM090A_FordMsg459BusHiSpd/15(GetTiSpan100MicroSec32bit)
  [SetNtcSts] -> MM090A_FordMsg459BusHiSpd/16(SetNtcSts)
  MM090A_FordMsg459BusHiSpd/1(FordVehTrlrAidAcqSts) -> [FordVehTrlrAidAcqSts]
  MM090A_FordMsg459BusHiSpd/2(FordVehTrlrAidHitchAg) -> [FordVehTrlrAidHitchAg]
  MM090A_FordMsg459BusHiSpd/3(FordVehTrlrAidHitchAgRate) -> [FordVehTrlrAidHitchAgRate]
  MM090A_FordMsg459BusHiSpd/4(FordVehTrlrAidIdnVal) -> [FordVehTrlrAidIdnVal]
  MM090A_FordMsg459BusHiSpd/5(FordVehTrlrAidTrakgSt) -> [FordVehTrlrAidTrakgSt]
  MM090A_FordMsg459BusHiSpd/6(FordVehTrlrAidTrlrRvsGuidcSts) -> [FordVehTrlrAidTrlrRvsGuidcSts]
  MM090A_FordMsg459BusHiSpd/7(FordVehTrlrBallToAxle) -> [FordVehTrlrBallToAxle]
  MM090A_FordMsg459BusHiSpd/8(FordVehTrlrHitchAgVld) -> [FordVehTrlrHitchAgVld]
  MM090A_FordMsg459BusHiSpd/9(FordVehTrlrHitchRateVld) -> [FordVehTrlrHitchRateVld]
  MM090A_FordMsg459BusHiSpd/10(FordVehTrlrTarVld) -> [FordVehTrlrTarVld]
  MM090A_FordMsg459BusHiSpd/11(FordVehTrlrTrakgStVld) -> [FordVehTrlrTrakgStVld]
  MM090A_FordMsg459BusHiSpd/12(TrlrAidStsThreePrsntInt) -> [TrlrAidStsThreePrsntInt]
  MM090A_FordMsg459BusHiSpd/13(ComIPduCallout_TrailerAidStat3_FD1) -> [ComIPduCallout_TrailerAidStat3_FD1]
  MM090A_FordMsg459BusHiSpd/14(ComTimeoutNotification_HitchToVehAxle_L_Calc) -> [ComTimeoutNotification_HitchToVehAxle_L_Calc]
  [ClrDiagcFlgProxy] -> MM086A_FordMsg443BusHiSpd/1(ClrDiagcFlgProxy)
  [FordCanDtcInhb] -> MM086A_FordMsg443BusHiSpd/2(FordCanDtcInhb)
  [FordEpsLifeCycMod] -> MM086A_FordMsg443BusHiSpd/3(FordEpsLifeCycMod)
  [FordTrlrBackupAssiEnad] -> MM086A_FordMsg443BusHiSpd/4(FordTrlrBackUpAssiEnad)
  TrlrLampCnnct_B_Actl/1 -> MM086A_FordMsg443BusHiSpd/5(Ford_TrlrLampCnnct_B_Actl1)
  [GetRefTmr100MicroSec32bit] -> MM086A_FordMsg443BusHiSpd/6(GetRefTmr100MicroSec32bit)
  [GetTiSpan100MicroSec32bit] -> MM086A_FordMsg443BusHiSpd/7(GetTiSpan100MicroSec32bit)
  [SetNtcSts] -> MM086A_FordMsg443BusHiSpd/8(SetNtcSts)
  MM086A_FordMsg443BusHiSpd/1(FordVehTrlrLampCnctnStsRaw) -> [FordVehTrlrLampCnctnStsRaw]
  MM086A_FordMsg443BusHiSpd/2(ComIPduCallout_TrailerInfo_FD1) -> [ComIPduCallout_TrailerInfo_FD1]
  MM086A_FordMsg443BusHiSpd/3(ComTimeoutNotification_TrlrLampCnnct_B_Actl) -> [ComTimeoutNotification_TrlrLampCnnct_B_Actl]
  [ClrDiagcFlgProxy] -> MM087A_FordMsg445BusHiSpd/1(ClrDiagcFlgProxy)
  [FordCanDtcInhb] -> MM087A_FordMsg445BusHiSpd/2(FordCanDtcInhb)
  [FordEpsLifeCycMod] -> MM087A_FordMsg445BusHiSpd/3(FordEpsLifeCycMod)
  [FordTrlrBackupAssiEnad] -> MM087A_FordMsg445BusHiSpd/4(FordTrlrBackUpAssiEnad)
  TrlrBrkActCnnct_B_Actl/1 -> MM087A_FordMsg445BusHiSpd/5(Ford_TrlrBrkActCnnct_B_Actl1)
  [GetRefTmr100MicroSec32bit] -> MM087A_FordMsg445BusHiSpd/6(GetRefTmr100MicroSec32bit)
  [GetTiSpan100MicroSec32bit] -> MM087A_FordMsg445BusHiSpd/7(GetTiSpan100MicroSec32bit)
  [SetNtcSts] -> MM087A_FordMsg445BusHiSpd/8(SetNtcSts)
  MM087A_FordMsg445BusHiSpd/1(FordVehTrlrBrkCnctnStsRaw) -> [FordVehTrlrBrkCnctnStsRaw]
  MM087A_FordMsg445BusHiSpd/2(ComIPduCallout_TrailerBrakeInfo_FD1) -> [ComIPduCallout_TrailerBrakeInfo_FD1]
  MM087A_FordMsg445BusHiSpd/3(ComTimeoutNotification_TrlrBrkActCnnct_B_Actl) -> [ComTimeoutNotification_TrlrBrkActCnnct_B_Actl]
  [ClrDiagcFlgProxy] -> MM069A_FordMsg3F1BusHiSpd/1(ClrDiagcFlgProxy)
  [FordCanDtcInhb] -> MM069A_FordMsg3F1BusHiSpd/2(FordCanDtcInhb)
  [FordEpsLifeCycMod] -> MM069A_FordMsg3F1BusHiSpd/3(FordEpsLifeCycMod)
  [FordMfgDiagcInhb] -> MM069A_FordMsg3F1BusHiSpd/4(FordMfgDiagcInhb)
  [FordMissMsgDiagcInhb] -> MM069A_FordMsg3F1BusHiSpd/5(FordMissMsgDiagcInhb)
  [FordTrlrBackupAssiEnad] -> MM069A_FordMsg3F1BusHiSpd/6(FordTrlrBackUpAssiEnad)
  TrlrAidCancl_B_Rq/1 -> MM069A_FordMsg3F1BusHiSpd/7(Ford_TrlrAidCancl_B_Rq1)
  [GetRefTmr100MicroSec32bit] -> MM069A_FordMsg3F1BusHiSpd/8(GetRefTmr100MicroSec32bit)
  [GetTiSpan100MicroSec32bit] -> MM069A_FordMsg3F1BusHiSpd/9(GetTiSpan100MicroSec32bit)
  [SetNtcSts] -> MM069A_FordMsg3F1BusHiSpd/10(SetNtcSts)
  MM069A_FordMsg3F1BusHiSpd/1(FordVehTrlrAidCnclReq) -> [FordVehTrlrAidCnclReq]
  MM069A_FordMsg3F1BusHiSpd/2(FordVehTrlrAidCnclReqVld) -> [FordVehTrlrAidCnclReqVld]
  MM069A_FordMsg3F1BusHiSpd/3(ComIPduCallout_APIM_Sen_Signals1_FD1) -> [ComIPduCallout_APIM_Sen_Signals1_FD1]
  MM069A_FordMsg3F1BusHiSpd/4(ComTimeoutNotification_TrlrAidCancl_B_Rq) -> [ComTimeoutNotification_TrlrAidCancl_B_Rq]
  [ClrDiagcFlgProxy] -> MM080A_FordMsg451BusHiSpd/1(ClrDiagcFlgProxy)
  [FordCanDtcInhb] -> MM080A_FordMsg451BusHiSpd/2(FordCanDtcInhb)
  [FordEpsLifeCycMod] -> MM080A_FordMsg451BusHiSpd/3(FordEpsLifeCycMod)
  [FordTrlrBackupAssiEnad] -> MM080A_FordMsg451BusHiSpd/4(FordTrlrBackupAssiEnad)
  TrlrRvrseEnbl_D2_Stat/1 -> MM080A_FordMsg451BusHiSpd/5(Ford_TrlrRvrseEnbl_D2_Stat1)
  TrlrRvrseMsgTxt_D2_Rq/1 -> MM080A_FordMsg451BusHiSpd/6(Ford_TrlrRvrseMsgTxt_D2_Rq)
  [GetRefTmr100MicroSec32bit] -> MM080A_FordMsg451BusHiSpd/7(GetRefTmr100MicroSec32bit)
  [GetTiSpan100MicroSec32bit] -> MM080A_FordMsg451BusHiSpd/8(GetTiSpan100MicroSec32bit)
  [SetNtcSts] -> MM080A_FordMsg451BusHiSpd/9(SetNtcSts)
  MM080A_FordMsg451BusHiSpd/1(FordVehTrlrRvsEnaRaw) -> [FordVehTrlrRvsEnaRaw]
  MM080A_FordMsg451BusHiSpd/2(FordVehTrlrRvsMsgTxtReqRaw) -> [FordVehTrlrRvsMsgTxtReqRaw]
  MM080A_FordMsg451BusHiSpd/3(ImgProcgDataPrsntInt) -> [ImgProcgDataPrsntInt]
  MM080A_FordMsg451BusHiSpd/4(ComIPduCallout_Image_Processing_Data_FD1) -> [ComIPduCallout_Image_Processing_Data_FD1]
  MM080A_FordMsg451BusHiSpd/5(ComTimeoutNotification_TrlrRvrseMsgTxt_D2_Rq) -> [ComTimeoutNotification_TrlrRvrseMsgTxt_D2_Rq]
  [ClrDiagcFlgProxy] -> MM092A_FordMsg47BusHiSpd/1(ClrDiagcFlgProxy)
  [FordCanDtcInhb] -> MM092A_FordMsg47BusHiSpd/2(FordCanDtcInhb)
  [FordEpsLifeCycMod] -> MM092A_FordMsg47BusHiSpd/3(FordEpsLifeCycMod)
  [FordTrlrBackupAssiEnad] -> MM092A_FordMsg47BusHiSpd/4(FordTrlrBackUpAssiEnad)
  TrlrAidCtl_U_RqDrv/1 -> MM092A_FordMsg47BusHiSpd/5(Ford_TrlrAidCtl_U_RqDrv1)
  TrlrAidSwtch_D_RqDrv/1 -> MM092A_FordMsg47BusHiSpd/6(Ford_TrlrAidSwtch_D_RqDrv)
  [GetRefTmr100MicroSec32bit] -> MM092A_FordMsg47BusHiSpd/7(GetRefTmr100MicroSec32bit)
  [GetTiSpan100MicroSec32bit] -> MM092A_FordMsg47BusHiSpd/8(GetTiSpan100MicroSec32bit)
  [SetNtcSts] -> MM092A_FordMsg47BusHiSpd/9(SetNtcSts)
  MM092A_FordMsg47BusHiSpd/1(FordVehTrlrAidKnobBtn) -> [FordVehTrlrAidKnobBtn]
  MM092A_FordMsg47BusHiSpd/2(FordVehTrlrAidKnobPosn) -> [FordVehTrlrAidKnobPosn]
  MM092A_FordMsg47BusHiSpd/3(ComIPduCallout_TrailerInfo_2_FD1) -> [ComIPduCallout_TrailerInfo_2_FD1]
  MM092A_FordMsg47BusHiSpd/4(ComTimeoutNotification_TrlrAidSwtch_D_RqDrv) -> [ComTimeoutNotification_TrlrAidSwtch_D_RqDrv]
  [ClrDiagcFlgProxy] -> MM088A_FordMsg45ABusHiSpd/1(ClrDiagcFlgProxy)
  [FordCanDtcInhb] -> MM088A_FordMsg45ABusHiSpd/2(FordCanDtcInhb)
  [FordEpsLifeCycMod] -> MM088A_FordMsg45ABusHiSpd/3(FordEpsLifeCycMod)
  [FordTrlrBackupAssiEnad] -> MM088A_FordMsg45ABusHiSpd/4(FordTrlrBackupAssiEnad)
  Ground/1 -> MM088A_FordMsg45ABusHiSpd/5(Ford_TrlrAnOffstDir_D_Mem1), MM088A_FordMsg45ABusHiSpd/6(Ford_TrlrAxleToBmpr_L_Actl), MM088A_FordMsg45ABusHiSpd/7(Ford_TrlrIdType_D_Stat1), MM088A_FordMsg45ABusHiSpd/8(Ford_TrlrId_No_Actl), MM088A_FordMsg45ABusHiSpd/9(Ford_TrlrRvrseCancl_B_Rq1)
  [GetRefTmr100MicroSec32bit] -> MM088A_FordMsg45ABusHiSpd/10(GetRefTmr100MicroSec32bit)
  [GetTiSpan100MicroSec32bit] -> MM088A_FordMsg45ABusHiSpd/11(GetTiSpan100MicroSec32bit)
  [SetNtcSts] -> MM088A_FordMsg45ABusHiSpd/12(SetNtcSts)
  MM088A_FordMsg45ABusHiSpd/1(FordVehTrlrAgOffsDirRaw) -> [FordVehTrlrAgOffsDirRaw]
  MM088A_FordMsg45ABusHiSpd/2(FordVehTrlrAidIdnNrRaw) -> [FordVehTrlrAidIdnNrRaw]
  MM088A_FordMsg45ABusHiSpd/3(FordVehTrlrAxleToBmpRaw) -> [FordVehTrlrAxleToBmpRaw]
  MM088A_FordMsg45ABusHiSpd/4(FordVehTrlrBackupAssiMeasVld) -> [FordVehTrlrBackupAssiMeasVld]
  MM088A_FordMsg45ABusHiSpd/5(FordVehTrlrIdnTypRaw) -> [FordVehTrlrIdnTypRaw]
  MM088A_FordMsg45ABusHiSpd/6(FordVehTrlrRvsCnclReqRaw) -> [FordVehTrlrRvsCnclReqRaw]
  MM088A_FordMsg45ABusHiSpd/7(TrlrAidDataPrsntInt) -> [TrlrAidDataPrsntInt]
  MM088A_FordMsg45ABusHiSpd/8(ComIPduCallout_TrailerAid_Data_FD1) -> [ComIPduCallout_TrailerAid_Data_FD1]
  MM088A_FordMsg45ABusHiSpd/9(ComTimeoutNotification_TrlrId_No_Actl) -> [ComTimeoutNotification_TrlrId_No_Actl]
  [ClrDiagcFlgProxy] -> MM083A_FordMsg457BusHiSpd/1(ClrDiagcFlgProxy)
  [FordCanDtcInhb] -> MM083A_FordMsg457BusHiSpd/2(FordCanDtcInhb)
  [FordEpsLifeCycMod] -> MM083A_FordMsg457BusHiSpd/3(FordEpsLifeCycMod)
  [FordTrlrBackupAssiEnad] -> MM083A_FordMsg457BusHiSpd/4(FordTrlrBackupAssiEnad)
  Ground22/1 -> MM083A_FordMsg457BusHiSpd/5(Ford_TrlrHitYaw_AnRate_Actl), MM083A_FordMsg457BusHiSpd/6(Ford_TrlrHitchYaw_An_Actl), MM083A_FordMsg457BusHiSpd/7(Ford_TrlrHitchYaw_D_Stat1), MM083A_FordMsg457BusHiSpd/8(Ford_TrlrYaw_W_Actl), MM083A_FordMsg457BusHiSpd/9(Ford_TrlrYaw_W_Actl_D_Qf1)
  [GetRefTmr100MicroSec32bit] -> MM083A_FordMsg457BusHiSpd/10(GetRefTmr100MicroSec32bit)
  [GetTiSpan100MicroSec32bit] -> MM083A_FordMsg457BusHiSpd/11(GetTiSpan100MicroSec32bit)
  [SetNtcSts] -> MM083A_FordMsg457BusHiSpd/12(SetNtcSts)
  MM083A_FordMsg457BusHiSpd/1(FordVehTrlrHitchAgRateRaw) -> [FordVehTrlrHitchAgRateRaw]
  MM083A_FordMsg457BusHiSpd/2(FordVehTrlrHitchYawAgRaw) -> [FordVehTrlrHitchYawAgRaw]
  MM083A_FordMsg457BusHiSpd/3(FordVehTrlrHitchYawSts) -> [FordVehTrlrHitchYawSts]
  MM083A_FordMsg457BusHiSpd/4(FordVehTrlrYawRateQlyFac) -> [FordVehTrlrYawRateQlyFac]
  MM083A_FordMsg457BusHiSpd/5(FordVehTrlrYawRateRaw) -> [FordVehTrlrYawRateRaw]
  MM083A_FordMsg457BusHiSpd/6(ComIPduCallout_TrailerAid_Stat2_FD1) -> [ComIPduCallout_TrailerAid_Stat2_FD1]
  MM083A_FordMsg457BusHiSpd/7(ComTimeoutNotification_TrlrHitchYaw_An_Actl) -> [ComTimeoutNotification_TrlrHitchYaw_An_Actl]
  [ClrDiagcFlgProxy] -> MM057A_FordMsg215BusHiSpd/1(ClrDiagcFlgProxy)
  [FordCanDtcInhb] -> MM057A_FordMsg215BusHiSpd/2(FordCanDtcInhb)
  [FordEpsLifeCycMod] -> MM057A_FordMsg215BusHiSpd/3(FordEpsLifeCycMod)
  [FordTrlrBackupAssiEnad] -> MM057A_FordMsg215BusHiSpd/4(FordTrlrBackupAssiEnad)
  Ground21/1 -> MM057A_FordMsg215BusHiSpd/5(Ford_TrlrAidMde_D_Rq1)
  [GetRefTmr100MicroSec32bit] -> MM057A_FordMsg215BusHiSpd/6(GetRefTmr100MicroSec32bit)
  [GetTiSpan100MicroSec32bit] -> MM057A_FordMsg215BusHiSpd/7(GetTiSpan100MicroSec32bit)
  [SetNtcSts] -> MM057A_FordMsg215BusHiSpd/8(SetNtcSts)
  MM057A_FordMsg215BusHiSpd/1(FordVehTrlrAidModReq) -> [FordVehTrlrAidModReq]
  MM057A_FordMsg215BusHiSpd/2(FordVehTrlrAidModReqVld) -> [FordVehTrlrAidModReqVld]
  MM057A_FordMsg215BusHiSpd/3(ComIPduCallout_APIM_Send_Signals_2_FD1) -> [ComIPduCallout_APIM_Send_Signals_2_FD1]
  MM057A_FordMsg215BusHiSpd/4(ComTimeoutNotification_TrlrAidMde_D_Rq) -> [ComTimeoutNotification_TrlrAidMde_D_Rq]

== system Ford_T3T6_ArchCnctnDigrm/Vehicle Com/Rx Messages/Transmission Data ==
  note: From COM
  note: From COM
  note: From COM
  GearLvrPos_D_Actl : Ground
  GearPos_D_Actl : Ground
  GearRvrse_D_Actl : Ground
  MM060A_FordMsg176BusHiSpd : Subsystem  Tag=0.0.X
      settings: AttributesFormatString=Version: %<Tag>
  MM061A_FordMsg202BusHiSpd : Subsystem  Tag=2.1.0  Description=The purpose of the Ford Message 202 Bus High Speed function is to provide the Electric Power Steering system with signal values for the vehicle speed, Torque Steer Compensation, Brake Pulse Reduction, Trailer Backup Assist functions from CAN. The Ford Message 202 function will perform the missing message and signal invalid diagnostics as well as provide a validity flag for the signal values and received message
      settings: AttributesFormatString=Version: %<Tag>
  MM066A_FordMsg230BusHiSpd : Subsystem  Tag=4.0.X  Description=The purpose of the Ford Message 230 Bus High Speed function is to provide the Electric Power Steering systemwith Trailer Back up Assist and Gear Lever Position signals from CAN. The Ford Message 230 function willperform the missing message and signal invalid diagnostics as well as provide a validity signal for the signalvalues and received message.
      settings: AttributesFormatString=Version: %<Tag>
  TrnRng_D_Rq : Ground
  VehVActlEng_D_Qf : Ground
  VehVActlEng_No_Cnt : Ground
  VehVActlEng_No_Cs : Ground
  VehVTrlrAid_B_Avail : Ground
  Veh_V_ActlEng : Ground
  tag scope: ComIPduCallout_EngVehicleSpThrottle2_HS2=global, ComIPduCallout_PowertrainData_10_FD1=global, ComIPduCallout_TransGearData_FD1=global, ComTimeoutNotification_Ford_VehVActlEng_D_Qf=global, ComTimeoutNotification_GearLvrPos_D_Actl=global, ComTimeoutNotification_GearPos_D_Actl=global, FordVehGearLvrPosn=global, FordVehGearLvrPosnVldInt=global, FordVehGearPosnRaw=global, FordVehGearPosnRawVldInt=global, FordVehGearRvsSts=global, FordVehGearRvsStsRaw=global, FordVehGearRvsStsVld=global, FordVehSpdChksEngModl=global, FordVehSpdCntrEngModl=global, FordVehSpdEngModl=global, FordVehSpdEngModlLoQlyVld=global, FordVehSpdEngModlRaw=global, FordVehSpdEngModlVld=global, FordVehSpdQlyFacEngModl=global, FordVehTrlrAidAvl=global, FordVehTrlrAidAvlRaw=global, FordVehTrlrBackupAssiAvlVld=global, FordVehTrsmDesGearRaw=global, FordVehTrsmDesGearRawVldInt=global
  wires:
  [ClrDiagcFlgProxy] -> MM061A_FordMsg202BusHiSpd/1(ClrDiagcFlgProxy)
  [FordAbsPrsnt] -> MM061A_FordMsg202BusHiSpd/2(FordAbsPrsnt)
  [FordBrkOscnRednEnad] -> MM061A_FordMsg202BusHiSpd/3(FordBrkOscnRednEnad)
  [FordCanDtcInhb] -> MM061A_FordMsg202BusHiSpd/4(FordCanDtcInhb)
  [FordEpsLifeCycMod] -> MM061A_FordMsg202BusHiSpd/5(FordEpsLifeCycMod)
  [FordInvldMsgDiagcInhb] -> MM061A_FordMsg202BusHiSpd/6(FordInvldMsgDiagcInhb)
  [FordMfgDiagcInhb] -> MM061A_FordMsg202BusHiSpd/7(FordMfgDiagcInhb)
  [FordMissMsgDiagcInhb] -> MM061A_FordMsg202BusHiSpd/8(FordMissMsgDiagcInhb)
  [FordTqSteerCmpEnad] -> MM061A_FordMsg202BusHiSpd/9(FordTqSteerCmpEnad)
  [FordTrlrBackupAssiEnad] -> MM061A_FordMsg202BusHiSpd/10(FordTrlrBackupAssiEnad)
  GearRvrse_D_Actl/1 -> MM061A_FordMsg202BusHiSpd/11(Ford_GearRvrse_D_Actl1)
  VehVActlEng_D_Qf/1 -> MM061A_FordMsg202BusHiSpd/12(Ford_VehVActlEng_D_Qf1)
  VehVActlEng_No_Cnt/1 -> MM061A_FordMsg202BusHiSpd/13(Ford_VehVActlEng_No_Cnt)
  VehVActlEng_No_Cs/1 -> MM061A_FordMsg202BusHiSpd/14(Ford_VehVActlEng_No_Cs)
  VehVTrlrAid_B_Avail/1 -> MM061A_FordMsg202BusHiSpd/15(Ford_VehVTrlrAid_B_Avail1)
  Veh_V_ActlEng/1 -> MM061A_FordMsg202BusHiSpd/16(Ford_Veh_V_ActlEng)
  [GetRefTmr100MicroSec32bit] -> MM061A_FordMsg202BusHiSpd/17(GetRefTmr100MicroSec32bit)
  [GetTiSpan100MicroSec32bit] -> MM061A_FordMsg202BusHiSpd/18(GetTiSpan100MicroSec32bit)
  [SetNtcSts] -> MM061A_FordMsg202BusHiSpd/19(SetNtcSts)
  MM061A_FordMsg202BusHiSpd/1(FordVehGearRvsSts) -> [FordVehGearRvsSts]
  MM061A_FordMsg202BusHiSpd/2(FordVehGearRvsStsRaw) -> [FordVehGearRvsStsRaw]
  MM061A_FordMsg202BusHiSpd/3(FordVehGearRvsStsVld) -> [FordVehGearRvsStsVld]
  MM061A_FordMsg202BusHiSpd/4(FordVehSpdChksEngModl) -> [FordVehSpdChksEngModl]
  MM061A_FordMsg202BusHiSpd/5(FordVehSpdCntrEngModl) -> [FordVehSpdCntrEngModl]
  MM061A_FordMsg202BusHiSpd/6(FordVehSpdEngModLoQlyVld) -> [FordVehSpdEngModlLoQlyVld]
  MM061A_FordMsg202BusHiSpd/7(FordVehSpdEngModl) -> [FordVehSpdEngModl]
  MM061A_FordMsg202BusHiSpd/8(FordVehSpdEngModlRaw) -> [FordVehSpdEngModlRaw]
  MM061A_FordMsg202BusHiSpd/9(FordVehSpdEngModlVld) -> [FordVehSpdEngModlVld]
  MM061A_FordMsg202BusHiSpd/10(FordVehSpdQlyFacEngModl) -> [FordVehSpdQlyFacEngModl]
  MM061A_FordMsg202BusHiSpd/11(FordVehTrlrAidAvl) -> [FordVehTrlrAidAvl]
  MM061A_FordMsg202BusHiSpd/12(FordVehTrlrAidAvlRaw) -> [FordVehTrlrAidAvlRaw]
  MM061A_FordMsg202BusHiSpd/13(FordVehTrlrBackupAssiAvlVld) -> [FordVehTrlrBackupAssiAvlVld]
  MM061A_FordMsg202BusHiSpd/14(ComIPduCallout_EngVehicleSpThrottle2_HS2) -> [ComIPduCallout_EngVehicleSpThrottle2_HS2]
  MM061A_FordMsg202BusHiSpd/15(ComTimeoutNotification_Ford_VehVActlEng_D_Qf) -> [ComTimeoutNotification_Ford_VehVActlEng_D_Qf]
  [ClrDiagcFlgProxy] -> MM060A_FordMsg176BusHiSpd/1(ClrDiagcFlgProxy)
  [FordCanDtcInhb] -> MM060A_FordMsg176BusHiSpd/2(FordCanDtcInhb)
  [FordEpsLifeCycMod] -> MM060A_FordMsg176BusHiSpd/3(FordEpsLifeCycMod)
  [FordInvldMsgDiagcInhb] -> MM060A_FordMsg176BusHiSpd/4(FordInvldMsgDiagcInhb)
  [FordMfgDiagcInhb] -> MM060A_FordMsg176BusHiSpd/5(FordMfgDiagcInhb)
  [FordMissMsgDiagcInhb] -> MM060A_FordMsg176BusHiSpd/6(FordMissMsgDiagcInhb)
  [FordTrlrBackupAssiEnad] -> MM060A_FordMsg176BusHiSpd/7(FordTrlrBackupAssiEnad)
  GearPos_D_Actl/1 -> MM060A_FordMsg176BusHiSpd/8(Ford_GearPos_D_Actl)
  [GetRefTmr100MicroSec32bit] -> MM060A_FordMsg176BusHiSpd/10(GetRefTmr100MicroSec32bit)
  [GetTiSpan100MicroSec32bit] -> MM060A_FordMsg176BusHiSpd/11(GetTiSpan100MicroSec32bit)
  [SetNtcSts] -> MM060A_FordMsg176BusHiSpd/12(SetNtcSts)
  MM060A_FordMsg176BusHiSpd/1(FordVehGearPosnRaw) -> [FordVehGearPosnRaw]
  MM060A_FordMsg176BusHiSpd/2(FordVehGearPosnRawVldInt) -> [FordVehGearPosnRawVldInt]
  MM060A_FordMsg176BusHiSpd/3(FordVehTrsmDesGearRaw) -> [FordVehTrsmDesGearRaw]
  MM060A_FordMsg176BusHiSpd/4(FordVehTrsmDesGearRawVldInt) -> [FordVehTrsmDesGearRawVldInt]
  MM060A_FordMsg176BusHiSpd/5(ComIPduCallout_PowertrainData_10_FD1) -> [ComIPduCallout_PowertrainData_10_FD1]
  MM060A_FordMsg176BusHiSpd/6(ComTimeoutNotification_GearPos_D_Actl) -> [ComTimeoutNotification_GearPos_D_Actl]
  TrnRng_D_Rq/1 -> MM060A_FordMsg176BusHiSpd/9(Ford_TrnRng_D_Rq)
  [ClrDiagcFlgProxy] -> MM066A_FordMsg230BusHiSpd/1(ClrDiagcFlgProxy)
  [FordCanDtcInhb] -> MM066A_FordMsg230BusHiSpd/2(FordCanDtcInhb)
  [FordEpsLifeCycMod] -> MM066A_FordMsg230BusHiSpd/3(FordEpsLifeCycMod)
  [FordTrlrBackupAssiEnad] -> MM066A_FordMsg230BusHiSpd/4(FordTrlrBackupAssiEnad)
  GearLvrPos_D_Actl/1 -> MM066A_FordMsg230BusHiSpd/5(Ford_GearLvrPos_D_Actl1)
  [GetRefTmr100MicroSec32bit] -> MM066A_FordMsg230BusHiSpd/6(GetRefTmr100MicroSec32bit)
  [GetTiSpan100MicroSec32bit] -> MM066A_FordMsg230BusHiSpd/7(GetTiSpan100MicroSec32bit)
  [SetNtcSts] -> MM066A_FordMsg230BusHiSpd/8(SetNtcSts)
  MM066A_FordMsg230BusHiSpd/1(FordVehGearLvrPosn) -> [FordVehGearLvrPosn]
  MM066A_FordMsg230BusHiSpd/2(FordVehGearLvrPosnVldInt) -> [FordVehGearLvrPosnVldInt]
  MM066A_FordMsg230BusHiSpd/3(ComIPduCallout_TransGearData_FD1) -> [ComIPduCallout_TransGearData_FD1]
  MM066A_FordMsg230BusHiSpd/4(ComTimeoutNotification_GearLvrPos_D_Actl) -> [ComTimeoutNotification_GearLvrPos_D_Actl]
